simulink model "Fadhlan_Firasyan_Mass_Spring_Damper_System_30Sep2024"  (R2023a)
settings: Solver=VariableStepAuto  StartTime=0.0  StopTime=10.0  RelTol=1e-3
undefined symbols (not defined in the file): c, dxdt_init, k, m, x_init
settings Model: Creator=HP  LastModifiedBy=HP

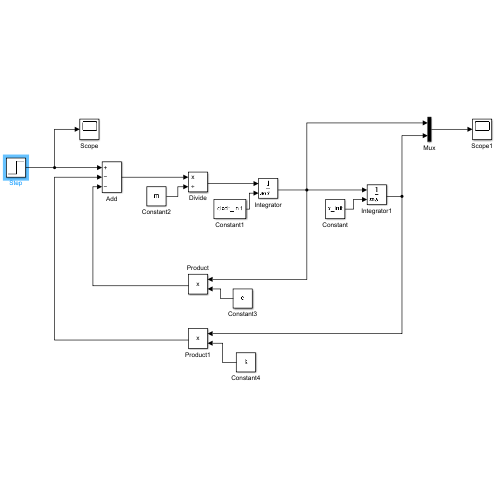
[thumbnail: Simulink's stored preview of the top-level diagram]
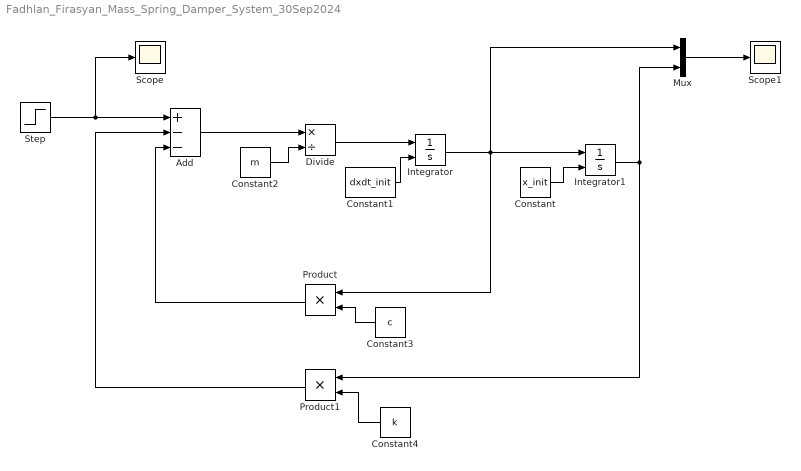
== system Fadhlan_Firasyan_Mass_Spring_Damper_System_30Sep2024 ==
  Add : Sum  Inputs=+--
  Constant : Constant  Value=x_init
  Constant1 : Constant  Value=dxdt_init
  Constant2 : Constant  Value=m
  Constant3 : Constant  Value=c
  Constant4 : Constant  Value=k
  Divide : Product  Inputs=*/
  Integrator : Integrator  InitialConditionSource=external
  Integrator1 : Integrator  InitialConditionSource=external
  Mux : Mux  Inputs=2
  Product : Product
  Product1 : Product
  Scope : Scope
  Scope1 : Scope
  Step : Step  SampleTime=0
  wires:
  Step/1 -> Scope/1, Add/1
  Divide/1 -> Integrator/1
  Integrator/1 -> Product/1, Integrator1/1, Mux/1
  Constant/1 -> Integrator1/2
  Constant2/1 -> Divide/2
  Constant3/1 -> Product/2
  Constant4/1 -> Product1/2
  Integrator1/1 -> Mux/2, Product1/1
  Mux/1 -> Scope1/1
  Product1/1 -> Add/2
  Product/1 -> Add/3
  Add/1 -> Divide/1
  Constant1/1 -> Integrator/2
